simulink model "qubeLQGR1"  (R2021b)
settings: Solver=ode1  StartTime=0.0  StopTime=50  RelTol=1e-3  EnableMultiTasking=on
values from neighbouring files (symbols this model uses):
  h = 0.01    [MPC_controller_testing.m]    (also in upright_LQR.m)
undefined symbols (not defined in the file or in its folder): Discrete, Humusoft, MF634, Time
libraries: sldrtlib x2, simulink x2, eeGeneralControl x2, ctrlSharedLib x1
settings Model: Creator=rbabuska  LastModifiedBy=wpanijhuis
settings SolverCC: AlgebraicLoopSolver=TrustRegion
settings DataIOCC: LimitDataPoints=on  SaveFormat=Array  SignalLoggingSaveFormat=ModelDataLogs  ReturnWorkspaceOutputs=off
settings OptimizationCC: ExpressionDepthLimit=2147483647  LifeSpan=inf
settings DebuggingCC: UnderspecifiedInitializationDetection=Classic  MergeDetectMultiDrivingBlocksExec=none  FcnCallInpInsideContextMsg=warning  StateNameClashWarn=warning  SFUnexpectedBacktrackingDiag=warning  SFNoUnconditionalDefaultTransitionDiag=warning  SFExecutionAtInitializationDiag=none  SFMachineParentedDataDiag=warning  ArithmeticOperatorsInVariantConditions=warning
settings HardwareCC: ProdBitPerPointer=32  ProdBitPerSizeT=32  ProdBitPerPtrDiffT=32  ProdLargestAtomicFloat=None  ProdIntDivRoundTo=Undefined  ProdEndianess=Unspecified  ProdWordSize=32  ProdHWDeviceType=32-bit Generic
settings ModelReferenceCC: PropagateSignalLabelsOutOfModel=off
settings SFSimCC: SimUseLocalCustomCode=off  CustomCodeUndefinedFunction=UseInterfaceOnly
settings RTWCC: RTWUseLocalCustomCode=off
settings CodeAppCC: StateflowObjectComments=on
settings GRTTargetCC: TargetLangStandard=C89/C90 (ANSI)  CombineOutputUpdateFcns=off  GRTInterface=on
settings ConfigComp: CovMetricSettings=dw  CovSaveCumulativeToWorkspaceVar=on  CovSaveSingleToWorkspaceVar=on  CovExternalEMLEnable=off  CovSFcnEnable=off

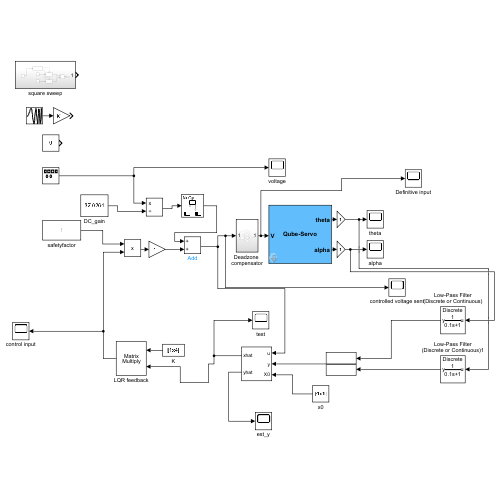
[thumbnail: Simulink's stored preview of the top-level diagram]
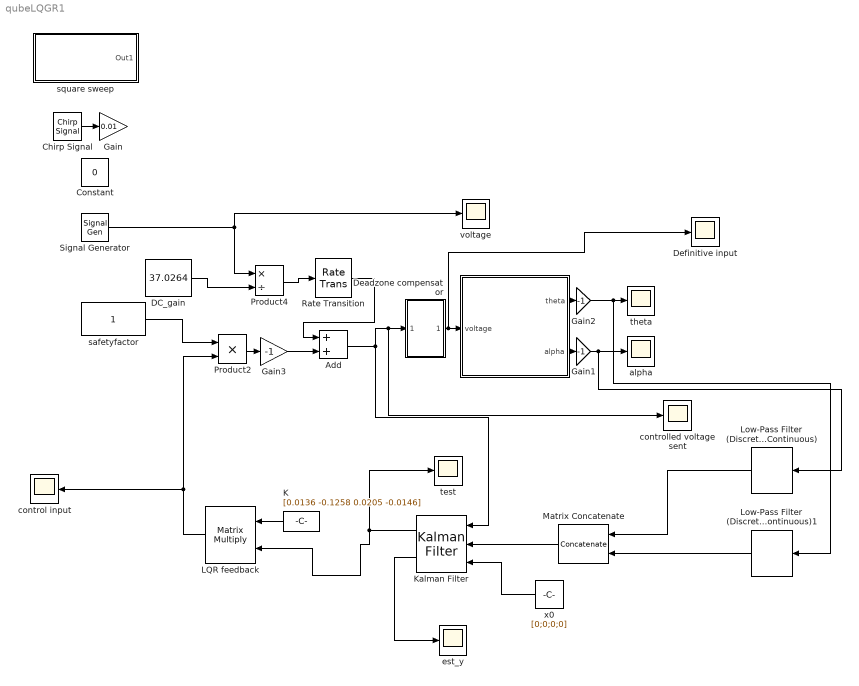
== system qubeLQGR1 ==
  " " : Subsystem  LoadFcn=hwinit  InitFcn=hwinit  mask{h=h}
      mask prompts: h "Sampling period [s]"
      mask Display:
      | disp('Qube-Servo')
      | port_label('output',1,'theta')
      | port_label('output',2,'alpha')
      | port_label('input',1,'V')
  Add : Sum  RndMeth=Nearest
  Chirp Signal : simulink/Sources/Chirp Signal  f1=4  T=50  f2=8
  Constant : Constant  Value=0
  DC_gain : Constant  Value=37.0264  SampleTime=h
  Deadzone compensator : Subsystem
  Definitive input : Scope
  Gain : Gain  Gain=0.01
  Gain1 : Gain  Gain=-1
  Gain2 : Gain  Gain=-1
  Gain3 : Gain  Gain=-1
  K : Constant  Value=[0.0136 -0.1258 0.0205 -0.0146]  VectorParams1D=off
  Kalman Filter : ctrlSharedLib/Kalman Filter  TimeDomain=Discrete-Time  UseCurrentEstimator=on  ModelSource=Individual A, B, C, D matrices  ModelSourceVariable=ss(0.95,1,1,0,1)  A=[0.9989,0.005179,0.009827,0.00005764;0.00111,0.9888,0.00005451,0.009913;-0.2085,1.025,0.9652,0.01317;0.2207,-2.237,0.01117,0.9788]  B=[0.06034;-0.05668;11.97;-11.27]  C=[1,0,0,0;0,1,0,0]  D=[0;0]  NumberOfStates=1  NumberOfInputs=1  NumberOfOutputs=1  InitialEstimateSource=Input port  X0=0  P0=10  UseK=off  UseGH=off  NumberOfProcessNoiseInputs=1  G=1  TimeInvariantG=on  H=0  TimeInvariantH=on  Q=6*1e-7  TimeInvariantQ=on  R=1e-10  TimeInvariantR=on  N=0  TimeInvariantN=on  AddInputPort=on  AddEnablePort=off  OutputEstimatedY=on  OutputP=off  Ts=h
  LQR feedback : Product  Multiplication=Matrix(*)
  Low-Pass Filter (Discrete or Continuous) : eeGeneralControl/Low-Pass Filter (Discrete or Continuous)  K=1  T=0.1  B=inf  A=-inf  init_option=Inherited from block input  x0=0  Ts=-1
  Low-Pass Filter (Discrete or Continuous)1 : eeGeneralControl/Low-Pass Filter (Discrete or Continuous)  K=1  T=0.1  B=inf  A=-inf  init_option=Inherited from block input  x0=0  Ts=-1
  Matrix Concatenate : Concatenate  ConcatenateDimension=2
  Product2 : Product
  Product4 : Product  Inputs=*/
  Rate Transition : RateTransition  OutPortSampleTime=h
  Signal Generator : SignalGenerator  WaveForm=square  Frequency=0.1
  alpha : Scope
  control input : Scope
  controlled voltage sent : Scope
  est_y : Scope
  safetyfactor : Constant
  square sweep : Subsystem
  test : Scope
  theta : Scope
  voltage : Scope
  x0 : Constant  Value=[0;0;0;0]
  wires:
  Gain2/1 -> Low-Pass Filter (Discrete or Continuous)1/1, theta/1
  Matrix Concatenate/1 -> Kalman Filter/2
  K/1 -> LQR feedback/1
  Kalman Filter/1 -> LQR feedback/2, test/1
  safetyfactor/1 -> Product2/1
  Kalman Filter/2 -> est_y/1
  LQR feedback/1 -> control input/1, Product2/2
  DC_gain/1 -> Product4/2
  Product4/1 -> Rate Transition/1
  Deadzone compensator/1(Out1) -> Definitive input/1, " "/1(voltage)
  Low-Pass Filter (Discrete or Continuous)/1 -> Matrix Concatenate/1
  Gain1/1 -> Low-Pass Filter (Discrete or Continuous)/1, alpha/1
  Low-Pass Filter (Discrete or Continuous)1/1 -> Matrix Concatenate/2
  Signal Generator/1 -> voltage/1, Product4/1
  " "/2(alpha) -> Gain1/1
  " "/1(theta) -> Gain2/1
  Add/1 -> Kalman Filter/1, controlled voltage sent/1, Deadzone compensator/1(In1)
  Chirp Signal/1 -> Gain/1
  x0/1 -> Kalman Filter/3
  Product2/1 -> Gain3/1
  Gain3/1 -> Add/2
  Rate Transition/1 -> Add/1

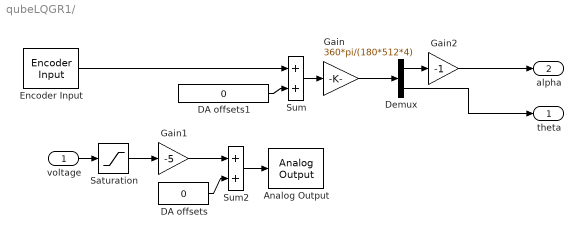
== system qubeLQGR1/  ==
  voltage : Inport
  Analog Output : sldrtlib/Analog Output  SampleTime=h  MaxMissedTicks=100  ShowMissedTicks=off  YieldWhenWaiting=off  DrvName=Humusoft/MF634  DrvAddress=4294967295  DrvOptions=0  Channels=[1]  RangeMode=2  VoltRange=1  InitialValue=0  FinalValue=0
      settings: AttributesFormatString=Humusoft\nMF634 [auto]
  DA offsets : Constant  Value=0
  DA offsets1 : Constant  Value=0  SampleTime=h
  Demux : Demux  Outputs=2
  Encoder Input : sldrtlib/Encoder Input  SampleTime=h  MaxMissedTicks=100  ShowMissedTicks=off  YieldWhenWaiting=off  DrvName=Humusoft/MF634  DrvAddress=4294967295  DrvOptions=0  Channels=[1,2]  QuadMode=3  IndexPulse=1  InputFilter=Inf  DataType=1
      settings: AttributesFormatString=Humusoft\nMF634 [auto]
  Gain : Gain  Gain=360*pi/(180*512*4)  SaturateOnIntegerOverflow=on  OutDataTypeStr=Inherit: Same as input  ParamDataTypeStr=Inherit: Same as input
  Gain1 : Gain  Gain=-5  SaturateOnIntegerOverflow=on  OutDataTypeStr=Inherit: Same as input  ParamDataTypeStr=Inherit: Same as input
  Gain2 : Gain  Gain=-1  SaturateOnIntegerOverflow=on  OutDataTypeStr=Inherit: Same as input  ParamDataTypeStr=Inherit: Same as input
  Saturation : Saturate  UpperLimit=1  LowerLimit=-1
  Sum : Sum  InputSameDT=on  SaturateOnIntegerOverflow=on  OutDataTypeStr=Inherit: Same as first input
  Sum2 : Sum  InputSameDT=on  SaturateOnIntegerOverflow=on  OutDataTypeStr=Inherit: Same as first input
  theta : Outport  Tag=Cable length
  alpha : Outport  Tag=Cable length  Port=2
  wires:
  Sum/1 -> Gain/1
  DA offsets1/1 -> Sum/2
  Gain1/1 -> Sum2/1
  Sum2/1 -> Analog Output/1
  DA offsets/1 -> Sum2/2
  voltage/1 -> Saturation/1
  Encoder Input/1 -> Sum/1
  Saturation/1 -> Gain1/1
  Demux/1 -> Gain2/1
  Gain/1 -> Demux/1
  Gain2/1 -> alpha/1
  Demux/2 -> theta/1

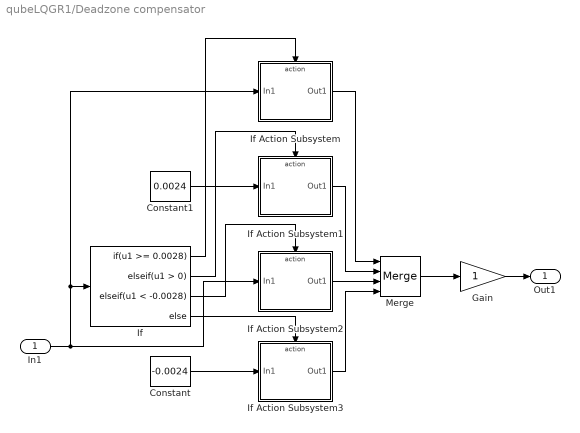
== system qubeLQGR1/Deadzone compensator ==
  In1 : Inport
  Constant : Constant  Value=-0.0024
  Constant1 : Constant  Value=0.0024
  Gain : Gain
  If : If  IfExpression=u1 >= 0.0028  ElseIfExpressions=u1 > 0, u1 < -0.0028
  If Action Subsystem : Subsystem  TreatAsAtomicUnit=on
  If Action Subsystem1 : Subsystem  TreatAsAtomicUnit=on
  If Action Subsystem2 : Subsystem  TreatAsAtomicUnit=on
  If Action Subsystem3 : Subsystem  TreatAsAtomicUnit=on
  Merge : Merge  Inputs=4
  Out1 : Outport
  wires:
  If Action Subsystem/1(Out1) -> Merge/1
  Gain/1 -> Out1/1
  If/4 -> If Action Subsystem3/Action
  If Action Subsystem2/1(Out1) -> Merge/3
  If/3 -> If Action Subsystem2/Action
  Merge/1 -> Gain/1
  If/2 -> If Action Subsystem1/Action
  Constant1/1 -> If Action Subsystem1/1(In1)
  If/1 -> If Action Subsystem/Action
  Constant/1 -> If Action Subsystem3/1(In1)
  If Action Subsystem3/1(Out1) -> Merge/4
  If Action Subsystem1/1(Out1) -> Merge/2
  In1/1 -> If Action Subsystem/1(In1), If/1, If Action Subsystem2/1(In1)

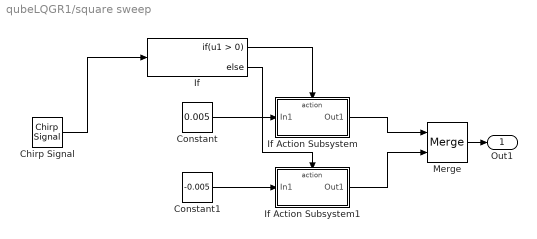
== system qubeLQGR1/square sweep ==
  Chirp Signal : simulink/Sources/Chirp Signal  f1=0  T=120  f2=5
  Constant : Constant  Value=0.005
  Constant1 : Constant  Value=-0.005
  If : If
  If Action Subsystem : Subsystem  TreatAsAtomicUnit=on
  If Action Subsystem1 : Subsystem  TreatAsAtomicUnit=on
  Merge : Merge
  Out1 : Outport
  wires:
  Merge/1 -> Out1/1
  If/2 -> If Action Subsystem1/Action
  Chirp Signal/1 -> If/1
  Constant/1 -> If Action Subsystem/1(In1)
  If Action Subsystem1/1(Out1) -> Merge/2
  If Action Subsystem/1(Out1) -> Merge/1
  If/1 -> If Action Subsystem/Action
  Constant1/1 -> If Action Subsystem1/1(In1)

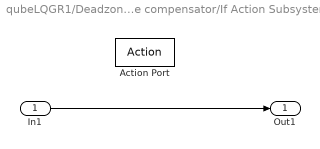
== system qubeLQGR1/Deadzone compensator/If Action Subsystem ==
  In1 : Inport
  Action Port : ActionPort  ActionPortLabel=if(u1 >= 0.0028)
  Out1 : Outport
  wires:
  In1/1 -> Out1/1

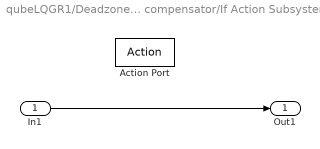
== system qubeLQGR1/Deadzone compensator/If Action Subsystem1 ==
  In1 : Inport
  Action Port : ActionPort  ActionPortLabel=elseif(u1 > 0)
  Out1 : Outport
  wires:
  In1/1 -> Out1/1

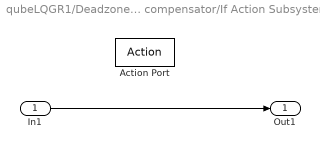
== system qubeLQGR1/Deadzone compensator/If Action Subsystem2 ==
  In1 : Inport
  Action Port : ActionPort  ActionPortLabel=elseif( u1 < -0.0028)
  Out1 : Outport
  wires:
  In1/1 -> Out1/1

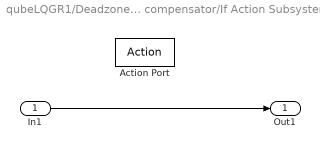
== system qubeLQGR1/Deadzone compensator/If Action Subsystem3 ==
  In1 : Inport
  Action Port : ActionPort  ActionPortLabel=else
  Out1 : Outport
  wires:
  In1/1 -> Out1/1

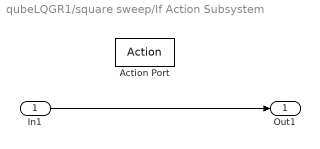
== system qubeLQGR1/square sweep/If Action Subsystem ==
  In1 : Inport
  Action Port : ActionPort  ActionPortLabel=if(u1 > 0)
  Out1 : Outport
  wires:
  In1/1 -> Out1/1

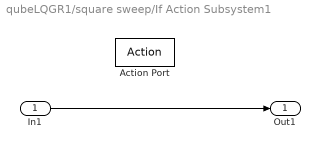
== system qubeLQGR1/square sweep/If Action Subsystem1 ==
  In1 : Inport
  Action Port : ActionPort  ActionPortLabel=else
  Out1 : Outport
  wires:
  In1/1 -> Out1/1
